simulink model "ControlBorroso"  (R2018b)
settings: Solver=VariableStepAuto  StartTime=0.0  StopTime=10.0  RelTol=1e-3
libraries: fuzblock x1
settings Model: Creator=marco  LastModifiedBy=marco

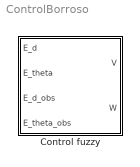
== system ControlBorroso ==
  Control fuzzy : Subsystem

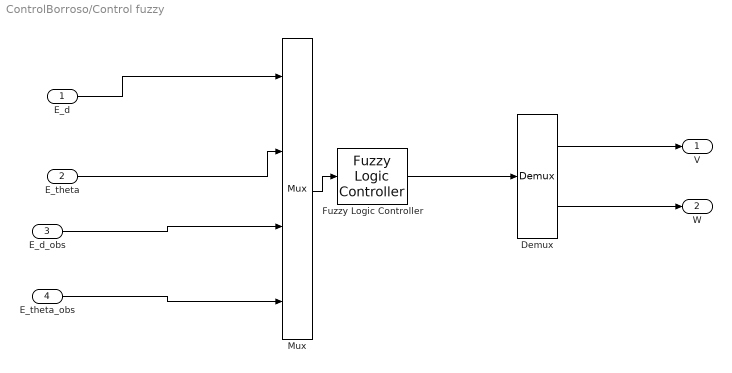
== system ControlBorroso/Control fuzzy ==
  "E_d " : Inport
  E_theta : Inport  Port=2
  E_d_obs : Inport  Port=3
  E_theta_obs : Inport  Port=4
  Demux : Demux  Outputs=2
  Fuzzy Logic Controller : fuzblock/Fuzzy Logic  Controller  FIS='ControlBorroso.fis'  OutputSampleNumber=101  DataType=double  FuzzifiedInputs=off  RuleFiringStrengths=off  RuleOutputs=off  AggregatedOutputs=off  SimulateUsing=Interpreted execution  OutOfRangeInputValueMessage=warning  NoRuleFiredMessage=warning  EmptyOutputFuzzySetMessage=warning
  Mux : Mux
  V : Outport
  "W " : Outport  Port=2
  wires:
  Mux/1 -> Fuzzy Logic Controller/1
  "E_d "/1 -> Mux/1
  Demux/1 -> V/1
  Demux/2 -> "W "/1
  E_theta/1 -> Mux/2
  Fuzzy Logic Controller/1 -> Demux/1
  E_d_obs/1 -> Mux/3
  E_theta_obs/1 -> Mux/4
